simulink model "EMobility_V9"  (R2023b)
settings: Solver=VariableStepAuto  StartTime=0.0  StopTime=10.0  RelTol=1e-3
undefined symbols (not defined in the file): Ion, Lithium
libraries: spsSeriesRLCBranchLib x19, spsIdealSwitchLib x13, spsCurrentMeasurementLib x8, spsIGBTDiodeLib x7, spsVoltageMeasurementLib x7, simulink x3, spsPLLLib x3, spsDiodeLib x2, spsPWMGenerator2LevelLib x2, spsPWMGeneratorDCDCLib x2, spsPowerLib x2, spsRMSLib x2
settings Model: Creator=valentinaribeiro  LastModifiedBy=gradykirsch

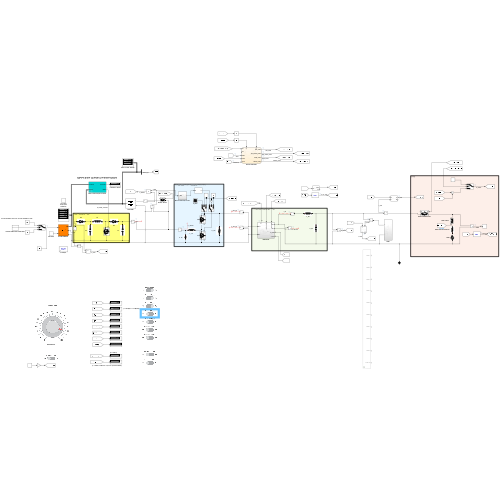
[thumbnail: Simulink's stored preview of the top-level diagram]
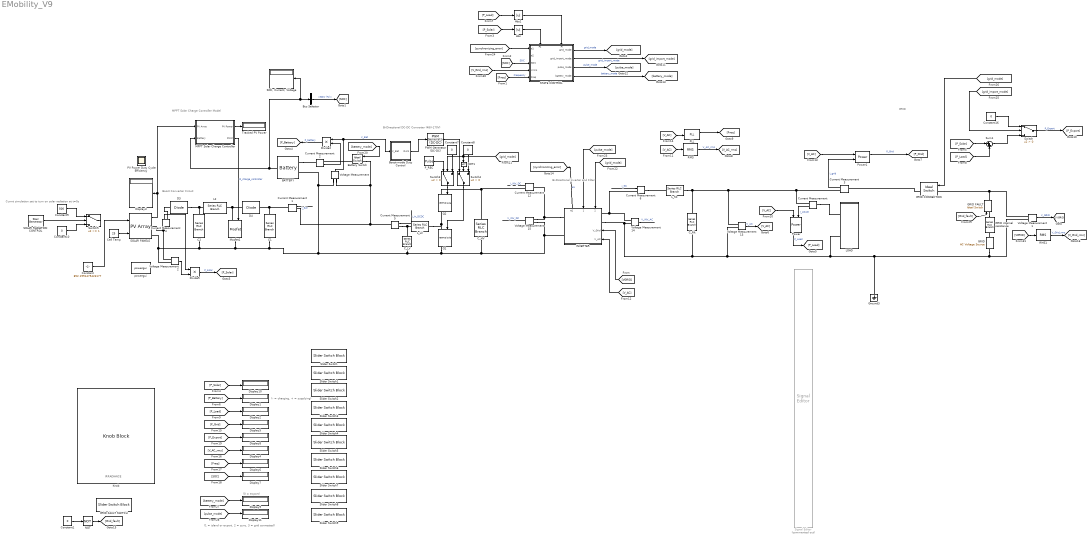
== system EMobility_V9 ==
  note: IRRADIANCE
  note: (- = charging, + = supplying)
  note: (0 = export)
  note: (1 = island or export, 2 = sync, 3 = grid connected)
  note: Bi-Directional Inverter and Filter
  note: GRID
  note: Boost Converter Circuit
  note: Bi-Directional DC-DC Converter (48V-170V)
  note: Currnt simulation set to turn on solar radiation at t=0s
  note: MPPT Solar Charge Controller Model
  " C1" : spsSeriesRLCBranchLib/Series RLC Branch  LConnTagsString=__new0  RConnTagsString=__new0  BranchType=C  Resistance=0.1  Inductance=1e-3  SetiL0=off  InitialCurrent=0  Capacitance=1  Setx0=off  InitialVoltage=0  Measurements=None
  Abs : Abs  SaturateOnIntegerOverflow=off
  Abs1 : Abs  SaturateOnIntegerOverflow=off
  BATTERY : spsBatteryLib/Battery  BatType=Lithium-Ion  ShowTempParam=off  ThermalPreset=no  ShowAgeParam=off  NomV=48  NomQ=80  SOC=89  Batt_Tr=30  PresetModel=on  MaxQ=80  MinV=36  FullV=55.8714  Dis_rate=34.7826  R=0.006  Normal_OP=72.3478  expZone="[51.8585      3.93043]"  current=[6.5 13 32.5]  Units=Time  Tci=20  NomT=20  T2=-30  MaxQ2=4.8  FullV2=7.1  Normal_OP2=5.655  expZone2="[6.58           1]"  Rca=0.6  ti=2000  Dp=0  Neq0=0  Tsim=1e6  Ta1=25  Qeol=5.4*0.9  Reol=0.013333*1.2  Char_age=[2.3478, 3]  Dis_age=[2.3478, 10]  N1=1500  N2=10500  N3=1000  N4=1400  Ta2=45  N5=950
      settings: LibrarySourceBlock=electricdrivelib/Extra Sources/Battery
  Battery Switch : spsIdealSwitchLib/Ideal Switch  Ron=0.001  Lon=0  IC=0  Rs=1e5  Cs=inf  Measurements=on
  Boost-mode Duty Control : Subsystem
  Bus Selector : BusSelector  OutputSignals=SOC (%)
  C2 : spsSeriesRLCBranchLib/Series RLC Branch  LConnTagsString=__new0  RConnTagsString=__new0  BranchType=C  Resistance=0.1  Inductance=1e-3  SetiL0=off  InitialCurrent=0  Capacitance=1000e-6  Setx0=off  InitialVoltage=0  Measurements=None
  C_HV : spsSeriesRLCBranchLib/Series RLC Branch  LConnTagsString=__new0  RConnTagsString=__new0  BranchType=C  Resistance=20  Inductance=159e-3  SetiL0=off  InitialCurrent=0  Capacitance=1.6e-3  Setx0=off  InitialVoltage=0  Measurements=None
  C_LV : spsSeriesRLCBranchLib/Series RLC Branch  LConnTagsString=__new0  RConnTagsString=__new0  BranchType=C  Resistance=20  Inductance=159e-3  SetiL0=off  InitialCurrent=0  Capacitance=0.5e-3  Setx0=off  InitialVoltage=0  Measurements=None
  C_filt : spsSeriesRLCBranchLib/Series RLC Branch  LConnTagsString=__new0  RConnTagsString=__new0  BranchType=C  Resistance=0  Inductance=1e-3  SetiL0=off  InitialCurrent=0  Capacitance=200e-6  Setx0=off  InitialVoltage=0  Measurements=None
  Cell Temp : Constant  Value=25
  Constant : Constant  Value=852.1991475423177
  Constant{1,7..8,10,16} (5 alike) : Constant  Value=0
  Constant9 : Constant  Value=500
  Current Measurement{,1..6,12} (8 alike) : spsCurrentMeasurementLib/Current Measurement  PhasorSimulation=off  OutputType=Complex  PSBequivalent=0
  D3 : spsDiodeLib/Diode  Ron=0.001  Lon=0  Vf=0.8  IC=0  UseSnubber=0  Rs=inf  Cs=0  Measurements=off
  D4 : spsDiodeLib/Diode  Ron=0.001  Lon=0  Vf=0.5  IC=0  UseSnubber=0  Rs=inf  Cs=0  Measurements=off
  Display{1..11} (11 alike) : Display
      Display7 settings: Decimation=1000
  Divide2 : Product  Inputs=**
  Divide5 : Product  Inputs=**
  GRID : spsACVoltageSourceLib/AC Voltage Source  Amplitude=170  Phase=0  Frequency=60  SampleTime=0  Measurements=None  BusType=swing  Pref=10e3  Qref=0  Qmin=-inf  Qmax=+inf
  GRID CONNECTION : spsIdealSwitchLib/Ideal Switch  Ron=0.001  Lon=0  IC=0  Rs=1e5  Cs=inf  Measurements=on
  GRID FAULT : spsIdealSwitchLib/Ideal Switch  Ron=0.001  Lon=0  IC=0  Rs=1e5  Cs=inf  Measurements=on
  GRID FAULT SWITCH : SliderSwitchBlock
      settings: Values={{'Off', 'On'}, [0 1]}
  GRID internal resistance : spsSeriesRLCBranchLib/Series RLC Branch  LConnTagsString=__new0  RConnTagsString=__new0  BranchType=R  Resistance=0.000001  Inductance=159e-3  SetiL0=off  InitialCurrent=0  Capacitance=100e-6  Setx0=off  InitialVoltage=0  Measurements=None
  Ground3 : spsGroundLib/Ground  LConnTagsString=a
  INVERTER : Subsystem
      settings: PortSchema="{\"entries\":[{\"content\":{\"sides\":[{\"content\":{\"connectorIds\":[\"LConn1\",\"LConn2\"]},\"type\":\"ConnectorPlacement.EquallySpacedRectSide\",\"uuid\":\"08b47f30-9f27-435b-83c4-c6fbe942e4e9\"},{\"content\":{\"connectorIds\":[\"RConn1\",\"RConn2\",\"In3\",\"In4\"],\"side\":\"RIGHT\"},\"type\":\"ConnectorPlacement.EquallySpacedRectSide\",\"uuid\":\"fbea0f57-7dc0-46de-be59-ba0dc15ef90e\"},{\"content\":{\"connectorIds\":[\"Out1\",\"In1\",\"In2\"],\"side\":\"TOP\"},\"type\":\"ConnectorPlacement.EquallySpacedRectSide\",\"uuid\":\"41f57134-76db-4888-b698-262c1208f49e\"}]},\"type\":\"ConnectorPlacement.EquallySpacedConnector\",\"uuid\":\"a2b9da51-a472-4525-b916-29c2121475f9\"}],\"packageUris\":[\"http://schema.mathworks.com/mf0/Connector/R2020b\"],\"version\":\"1.0\"}"
  Knob : KnobBlock  ScaleMax=1000
  L2 : spsSeriesRLCBranchLib/Series RLC Branch  LConnTagsString=__new0  RConnTagsString=__new0  BranchType=L  Resistance=1  Inductance=0.01  SetiL0=off  InitialCurrent=0  Capacitance=1e-6  Setx0=off  InitialVoltage=0  Measurements=None
  LOAD : Subsystem
  L_LV : spsSeriesRLCBranchLib/Series RLC Branch  LConnTagsString=__new0  RConnTagsString=__new0  BranchType=L  Resistance=0  Inductance=0.003  SetiL0=off  InitialCurrent=0  Capacitance=100e-6  Setx0=off  InitialVoltage=0  Measurements=None
  L_filt : spsSeriesRLCBranchLib/Series RLC Branch  LConnTagsString=__new0  RConnTagsString=__new0  BranchType=L  Resistance=0  Inductance=0.003  SetiL0=off  InitialCurrent=0  Capacitance=100e-6  Setx0=off  InitialVoltage=0  Measurements=None
  MPPT Solar Charge Controller : Subsystem  mask(MPPT Solar Charge Controller Block){dD=1e-6, BattCV=55.4, Fsw=1000}
      mask prompts: dD "MPPT Duty Cycle (delta) Step Size"; BattCV "Battery Charging Constant Voltage (V)"; Fsw "PWM Switching frequency (Hz):"
      mask help:
      | MPPT Solar Charge Controller Block
      | Developed by Rodney Tan (PhD)
      | Version 1.00 Oct 2019
      |
      | This block perform solar photovoltaic Maximum Power Point Tracking based on Perturbation & Observation algorithm and charge lead acid battery using three stage charging algorithm.
      mask Help:
      | <b><u>Block Setting</u></b>
      | 
      | <b>MPPT Duty Cycle Step Size</b>
      | Specify the MPPT duty cycle (delta) step size. Default value is 1e-5.
      | 
      | <b>Battery Charging Constant Voltage (V)</b>
      | Specify the battery charging constant voltage for absorption stage.
      | 
      | <b>PWM Switching Frequency (Hz)</b>
      | Specify the PWM switching frequency in Hz.
      mask TypeOptions Fsw:
      | PWM Generator
      | (DC-DC)/Fsw
  Mosfet1 : spsMosfetLib/Mosfet  Ron=0.02  Lon=0  Rd=0.01  Vfd=0  IC=0  Rs=1e5  Cs=inf  Measurements=off
  NOT : Logic  Operator=NOT  IconShape=distinctive  AllPortsSameDT=off  OutDataTypeStr=boolean
  NOT1 : Logic  Operator=NOT  IconShape=distinctive  AllPortsSameDT=off  OutDataTypeStr=boolean
  PLL : spsPLLLib/PLL  Fmin=45  Par_Init=[0, 60]  ParK=[180, 3200, 1]  TcD=1e-4  MaxRateChangeFreq=12  FilterCutOffFreq=25  Ts=0  AGC=on
      settings: LibrarySourceBlock=sps_lib/Control/PLL
  PV Power Duty Cycle Efficiency : Scope
      settings: Floating=on
  PWM Generator (DC-DC) : spsPWMGeneratorDCDCLib/PWM Generator (DC-DC)  Fsw=5000  Ts=0
  P_REC : DiscretePulseGenerator  PulseType=Time based  Period=1/5000  PulseWidth=26
  Power : spsPowerLib/Power  Freq=60  Vinit=[1, 0]  Iinit=[1, 0]  Ts=0
  Power1 : spsPowerLib/Power  Freq=60  Vinit=[1, 0]  Iinit=[1, 0]  Ts=0
  Q1 : spsIGBTDiodeLib/IGBT//Diode  Ron=1e-3  Rs=1e5  Cs=inf  Measurements=on
  Q2 : spsIGBTDiodeLib/IGBT//Diode  Ron=1e-3  Rs=1e5  Cs=inf  Measurements=on
  RMS : spsRMSLib/RMS  TrueRMS=on  Freq=60  RMSInit=120  Ts=0
  RMS1 : spsRMSLib/RMS  TrueRMS=on  Freq=60  RMSInit=120  Ts=0
  "SOC, Current, Voltage" : Display
  SOLAR PANELS : spsPVArrayLib/PV Array  Npar=8  Nser=10  PlotType=array @ 25 deg.C & specified irradiances  S_vec="[ 1000  800  600 400 200 ]"  Temp_C_vec="[ 45 25  ]"  ModuleName=Tesla Inc. SR24S3-2  PlotWhenSelected=off  Pm=23.4  Ncell=6  Voc=3.8  Isc=8.35  Vm=3  Im=7.8  beta_Voc_pc=-0.325  alpha_Isc_pc=0.048  beta_Voc=-0.01235  alpha_Isc=0.004008  IL=8.3755  I0=7.7166e-11  nI=0.97085  Rsh=23.4287  Rs=0.046227  RobustModel=off  RobustCellTemperature=313.3991  BAL=off  Tc=1e-6  Tfilter=1e-5
  SOLAR RADIATION CONTROL : spsStairGeneratorLib/Stair Generator  t=[0, 0.2, 0.4]  e=[1, 1, 1]  Ts=0
  STATE CONTROL : Stateflow chart  TreatAsAtomicUnit=on
      settings: PortSchema="{\"entries\":[{\"content\":{\"sides\":[{\"content\":{\"connectorIds\":[\"In3\",\"In5\",\"In6\",\"In4\",\"In7\"]},\"type\":\"ConnectorPlacement.EquallySpacedRectSide\",\"uuid\":\"b48b8e79-9223-4f44-9ca2-01abafb2610b\"},{\"content\":{\"connectorIds\":[\"Out1\",\"Out2\",\"Out3\",\"Out4\"],\"side\":\"RIGHT\"},\"type\":\"ConnectorPlacement.EquallySpacedRectSide\",\"uuid\":\"69043a30-cfac-4fa3-beb1-dafea7c61121\"},{\"content\":{\"connectorIds\":[\"In1\",\"In2\"],\"side\":\"TOP\"},\"type\":\"ConnectorPlacement.EquallySpacedRectSide\",\"uuid\":\"c5081c87-0412-4df0-923f-4518851b42d3\"}]},\"type\":\"ConnectorPlacement.EquallySpacedConnector\",\"uuid\":\"4eeccdef-121a-476a-b6e9-b0cda67e3776\"}],\"packageUris\":[\"http://schema.mathworks.com/mf0/Connector/R2020b\"],\"version\":\"1.0\"}"
  Signal Editor : SignalEditorBlockLib/Signal Editor  Commented=on  FileName=/Volumes/Extreme_SSD/MATLAB/loadsignal.mat  ActiveScenario=Scenario  ActiveSignal=Load 1  IsBus=off  OutputBusObjectStr=Bus: BusObject  SampleTime=0  Interpolate=off  ZeroCross=off  OutputAfterFinalValue=Setting to zero  Unit=inherit  PreserveSignalName=on  ApplySigPropsToAllScenarios=on  ApplySigPropsToAllSignals=off
  Slider Switch{,1..9} (10 alike) : SliderSwitchBlock
      settings: Values={{'Off', 'On'}, [0 1]}
  Sum1 : Sum  Inputs=|++
  Switch : Switch  Criteria=u2 > Threshold  SaturateOnIntegerOverflow=off  InputSameDT=off
  Switch3 : Switch  Criteria=u2 > Threshold  SaturateOnIntegerOverflow=off  InputSameDT=off
  Switch4 : Switch  Criteria=u2 > Threshold  SaturateOnIntegerOverflow=off  InputSameDT=off
  Switch5 : Switch  Threshold=1  SaturateOnIntegerOverflow=off  InputSameDT=off
  Tracked PV Power : Display
  Voltage Measurement{,1..2,13..15} (6 alike) : spsVoltageMeasurementLib/Voltage Measurement  PhasorSimulation=off  OutputType=Complex  PSBequivalent=0
  powergui : sps_lib/powergui  Priority=1  SimulationMode=Discrete  SampleTime=1/1e5  frequency=60  Iterations=50  frequencyindice=0  Pbase=100e6  ErrMax=1e-4  UnitsV=kV  UnitsW=MW  buscounter=0  FunctionMessages=off  echomessages=off  EnableUseOfTLC=off  CurrentSourceSwitches=off  DisableSnubberDevices=off  DisableRonSwitches=off  DisableVfSwitches=off  DisplayEquations=off  AutomaticDiscreteSolvers=off  SolverType=Tustin/Backward Euler (TBE)  Interpol=off  ExternalGateDelay=off  methode=off  Ts=100  x0status=blocks  SPID=off  SwTol=0  HookPort=off  NonlinearTolerance=1e-4  nMaxIteration=100  ContinueOnMaxIteration=off  RestoreLinks=warning  ResistiveCurrentMeasurement=off  Frange=[0:2:500]  Ylog=off  Xlog=on  ShowGrid=off  save=off  variable=ZData  structure=0  ZoomFFT=off  StartTime=0.0  cycles=1  DisplayStyle=1  fundamental=60  FreqAxis=off  MaxFrequency=1000  frequencyindicesteady=1  RmsSteady=1  display=off
  wires:
  Voltage Measurement15/1 -> ?  "V_INV_DC"
  SOLAR PANELS/1 -> MPPT Solar Charge Controller/1(PV Array), Display3/1
  RMS/1 -> [V_AC_rms]  "V_AC_rms"
  INVERTER/1(e1) -> [synchronizing_error]  "e1"
  Divide2/1 -> [P_Battery]  "P_battery"
  P_REC/1 -> Switch3/1
  NOT1/1 -> Switch4/2
  Current Measurement/1 -> Power/2  "I_LOAD"
  Voltage Measurement14/1 -> ?  "V_INV_AC"
  STATE CONTROL/3(pulse_mode) -> [pulse_mode]  "pulse_mode"
  Voltage Measurement13/1 -> [V_AC]  "V_AC"
  Current Measurement2/1 -> Divide2/2
  Constant7/1 -> Switch3/3
  Voltage Measurement1/1 -> [VGRID]  "V_GRID"
  BATTERY/1 -> Bus Selector/1, "SOC, Current, Voltage"/1, MPPT Solar Charge Controller/2(Battery)
  Constant10/1 -> Switch5/3
  SOLAR RADIATION CONTROL/1 -> Switch5/2
  Switch3/1 -> Q2/1
  Switch4/1 -> Q1/1
  PWM Generator (DC-DC)/1 -> Switch4/1
  MPPT Solar Charge Controller/1(PV Power) -> Tracked PV Power/1
  Cell Temp/1 -> SOLAR PANELS/2
  MPPT Solar Charge Controller/2(PWM) -> Mosfet1/1  "D_charge_controller"
  Current Measurement12/1 -> ?  "I_INV_DC"
  Constant9/1 -> Switch5/1
  PLL/1 -> [Freq]
  Voltage Measurement/1 -> Divide2/1, Boost-mode Duty Control/1(V_Bat)  "V_Bat"
  [VGRID] -> INVERTER/3(V_Grid)
  Constant8/1 -> Switch4/3
  STATE CONTROL/1(grid_mode) -> [grid_mode]  "grid_mode"
  Bus Selector/1 -> [SOC]  "<SOC (%)>"
  Current Measurement3/1 -> Power1/2  "I_grid"
  Divide5/1 -> [P_Solar]  "P_solar"
  Voltage Measurement2/1 -> Divide5/2
  Current Measurement4/1 -> Divide5/1
  Abs1/1 -> STATE CONTROL/2(Pl)
  Abs/1 -> STATE CONTROL/1(Ps)
  Power1/1 -> [P_Grid]  "P_Grid"
  Power/1 -> [P_Load]  "P_Load"
  STATE CONTROL/4(battery_mode) -> [battery_mode]  "battery_mode"
  STATE CONTROL/2(grid_import_mode) -> [grid_import_mode]  "grid_import_mode"
  Current Measurement5/1 -> ?  "i_in_DCDC"
  Current Measurement6/1 -> ?  "I_filt"
  Switch/1 -> [P_Export]  "P_Export"
  Sum1/1 -> Switch/3
  Constant16/1 -> Switch/1
  [P_Solar] -> Abs/1
  [P_Solar] -> Display10/1
  [P_Solar] -> Sum1/1
  Boost-mode Duty Control/1(Out1) -> PWM Generator (DC-DC)/1
  Current Measurement1/1 -> ?  "I_Sun"
  [P_Battery] -> Display1/1
  [P_Load] -> Abs1/1
  [P_Load] -> Sum1/2
  [P_Load] -> Display2/1
  [V_AC] -> Power/1
  [V_AC] -> RMS/1
  [V_AC] -> INVERTER/4(V_AC)
  [V_AC] -> Power1/1
  [V_AC] -> PLL/1
  [P_Grid] -> Display5/1
  [Freq] -> Display6/1
  [V_AC_rms] -> Display4/1
  [Freq] -> STATE CONTROL/7(Freq)  "Frequency"
  [SOC] -> STATE CONTROL/6(SOC)  "SOC"
  [SOC] -> Display7/1
  [P_Export] -> Display8/1
  [battery_mode] -> Battery Switch/1
  [grid_mode] -> NOT1/1, Switch3/2
  [grid_mode] -> INVERTER/2(grid_mode)
  [pulse_mode] -> INVERTER/1(pulse_mode)
  [synchronizing_error] -> STATE CONTROL/3(e1)
  [grid_import_mode] -> Switch/2
  [grid_mode] -> GRID CONNECTION/1
  [pulse_mode] -> Display11/1
  [battery_mode] -> Display9/1
  Constant/1 -> SOLAR PANELS/1
  [Grid_fault] -> GRID FAULT/1
  Constant1/1 -> NOT/1
  NOT/1 -> [Grid_fault]
  [V_Grid_rms] -> STATE CONTROL/4(Vrms)
  RMS1/1 -> [V_Grid_rms]  "V_Grid_rms"
  [VGRID] -> RMS1/1
  connections:
  C_LV/RConn1 -- Voltage Measurement/LConn2 -- BATTERY/LConn2 -- " C1"/RConn1 -- Mosfet1/RConn1 -- SOLAR PANELS/RConn2 -- Voltage Measurement2/LConn2 -- C2/RConn1 -- Q1/RConn1 -- C_HV/RConn1 -- Voltage Measurement15/LConn2 -- INVERTER/LConn2
  Current Measurement1/RConn1 -- Battery Switch/LConn1 -- Voltage Measurement/LConn1 -- Current Measurement5/LConn1
  Voltage Measurement1/LConn1 -- GRID FAULT/RConn1 -- GRID CONNECTION/LConn1
  L2/LConn1 -- C2/LConn1 -- D3/RConn1
  L_filt/RConn1 -- Current Measurement/RConn1 -- Current Measurement3/RConn1 -- Voltage Measurement13/LConn1 -- C_filt/LConn1
  Voltage Measurement13/LConn2 -- GRID/LConn1 -- Voltage Measurement1/LConn2 -- Ground3/LConn1 -- LOAD/LConn2 -- INVERTER/RConn2 -- Voltage Measurement14/LConn2 -- C_filt/RConn1
  INVERTER/LConn1 -- Current Measurement12/LConn1 -- Voltage Measurement15/LConn1
  L_LV/RConn1 -- Q2/RConn1 -- Q1/LConn1
  Mosfet1/LConn1 -- L2/RConn1 -- D4/LConn1
  C_HV/LConn1 -- Q2/LConn1 -- Current Measurement12/RConn1
  Voltage Measurement14/LConn1 -- Current Measurement6/RConn1 -- INVERTER/RConn1
  GRID/RConn1 -- GRID internal resistance/LConn1
  BATTERY/LConn1 -- Current Measurement2/LConn1
  GRID CONNECTION/RConn1 -- Current Measurement3/LConn1
  " C1"/LConn1 -- Current Measurement1/LConn1 -- D4/RConn1
  Current Measurement4/LConn1 -- Voltage Measurement2/LConn1 -- SOLAR PANELS/RConn1
  D3/LConn1 -- Current Measurement4/RConn1
  Battery Switch/RConn1 -- Current Measurement2/RConn1
  L_LV/LConn1 -- Current Measurement5/RConn1 -- C_LV/LConn1
  Current Measurement6/LConn1 -- L_filt/LConn1
  Current Measurement/LConn1 -- LOAD/LConn1
  GRID FAULT/LConn1 -- GRID internal resistance/RConn1

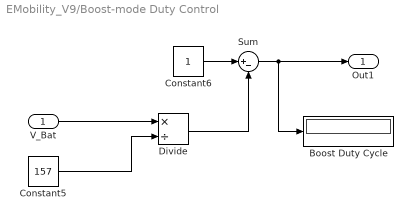
== system EMobility_V9/Boost-mode Duty Control ==
  V_Bat : Inport
  Boost Duty Cycle : Display
  Constant5 : Constant  Value=157
  Constant6 : Constant
  Divide : Product  Inputs=*/
  Sum : Sum  Inputs=|+-
  Out1 : Outport
  wires:
  Divide/1 -> Sum/2
  Constant6/1 -> Sum/1
  V_Bat/1 -> Divide/1
  Constant5/1 -> Divide/2
  Sum/1 -> Out1/1, Boost Duty Cycle/1

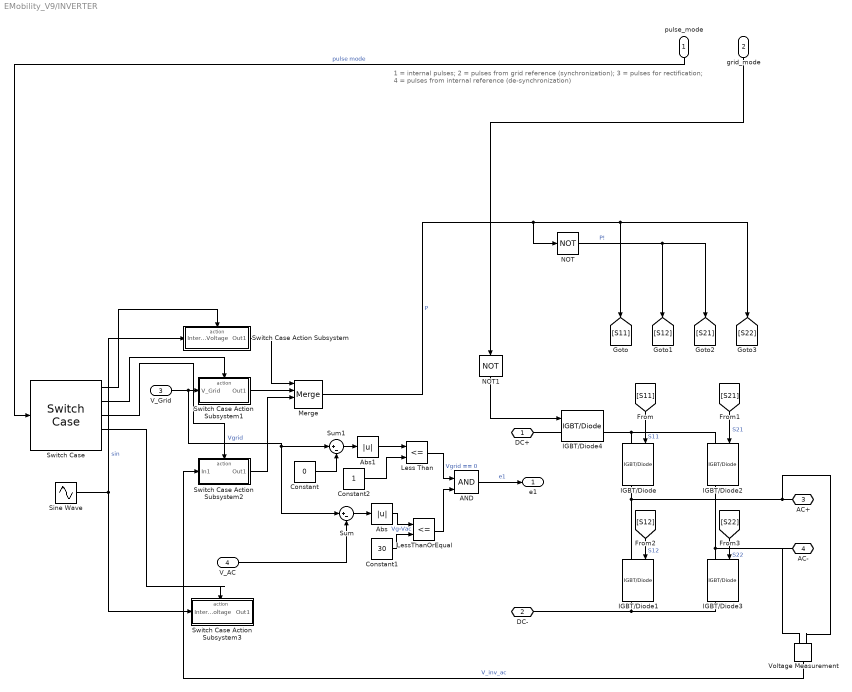
== system EMobility_V9/INVERTER ==
  note: 1 = internal pulses; 2 = pulses from grid reference (synchronization); 3 = pulses for rectification; 4 = pulses from internal reference (de-synchronization)
  pulse_mode : Inport
  grid_mode : Inport  Port=2
  V_Grid : Inport  Port=3
  V_AC : Inport  Port=4
  AND : Logic  IconShape=distinctive  AllPortsSameDT=off  OutDataTypeStr=boolean
  Abs : Abs  SaturateOnIntegerOverflow=off
  Abs1 : Abs  SaturateOnIntegerOverflow=off
  Constant : Constant  Value=0
  Constant1 : Constant  Value=30
  Constant2 : Constant
  IGBT/Diode{,1..4} (5 alike) : spsIGBTDiodeLib/IGBT//Diode  Ron=1e-3  Rs=1e5  Cs=inf  Measurements=on
  Less Than : RelationalOperator  Operator=<=  OutDataTypeStr=boolean  RndMeth=Simplest  InputSameDT=off
  LessThanOrEqual : RelationalOperator  Operator=<=  OutDataTypeStr=boolean  RndMeth=Simplest  InputSameDT=off
  Merge : Merge  Inputs=4
  NOT : Logic  Operator=NOT  IconShape=distinctive  AllPortsSameDT=off  OutDataTypeStr=boolean
  NOT1 : Logic  Operator=NOT  IconShape=distinctive  AllPortsSameDT=off  OutDataTypeStr=boolean
  Sine Wave : Sin  Frequency=60*2*pi  Phase=pi/2  SampleTime=0
  Sum : Sum  Inputs=|+-
  Sum1 : Sum  Inputs=|+-
  Switch Case : SwitchCase  CaseConditions={1,2,3,4}
  Switch Case Action Subsystem : Subsystem  TreatAsAtomicUnit=on
  Switch Case Action Subsystem1 : Subsystem  TreatAsAtomicUnit=on
  Switch Case Action Subsystem2 : Subsystem  TreatAsAtomicUnit=on
  Switch Case Action Subsystem3 : Subsystem  TreatAsAtomicUnit=on
  Voltage Measurement : spsVoltageMeasurementLib/Voltage Measurement  PhasorSimulation=off  OutputType=Complex  PSBequivalent=0
  DC+ : PMIOPort  Side=Left
  DC- : PMIOPort  Port=2  Side=Left
  AC+ : PMIOPort  Port=3  Side=Right
  AC- : PMIOPort  Port=4  Side=Right
  e1 : Outport
  wires:
  [S11] -> IGBT/Diode/1  "S11"
  [S21] -> IGBT/Diode2/1  "S21"
  [S12] -> IGBT/Diode1/1  "S12"
  [S22] -> IGBT/Diode3/1  "S22"
  Merge/1 -> NOT/1, [S11], [S22]  "P"
  NOT/1 -> [S21], [S12]  "P!"
  Voltage Measurement/1 -> Switch Case Action Subsystem2/1(In1)  "V_inv_ac"
  pulse_mode/1 -> Switch Case/1  "pulse mode"
  NOT1/1 -> IGBT/Diode4/1
  V_Grid/1 -> Sum1/1, Sum/1, Switch Case Action Subsystem1/1(V_Grid)  "Vgrid"
  Switch Case/1 -> Switch Case Action Subsystem/Action
  Switch Case/2 -> Switch Case Action Subsystem1/Action
  Switch Case/3 -> Switch Case Action Subsystem2/Action
  Switch Case Action Subsystem/1(Out1) -> Merge/1
  Switch Case Action Subsystem1/1(Out1) -> Merge/2
  Switch Case Action Subsystem2/1(Out1) -> Merge/3
  grid_mode/1 -> NOT1/1
  Sum/1 -> Abs/1
  Less Than/1 -> AND/1  "Vgrid == 0"
  AND/1 -> e1/1  "e1"
  Abs/1 -> LessThanOrEqual/1  "Vg-Vac"
  Constant1/1 -> LessThanOrEqual/2
  LessThanOrEqual/1 -> AND/2
  Constant/1 -> Sum1/2
  Constant2/1 -> Less Than/2
  Sum1/1 -> Abs1/1
  Abs1/1 -> Less Than/1
  V_AC/1 -> Sum/2
  Switch Case/4 -> Switch Case Action Subsystem3/Action
  Sine Wave/1 -> Switch Case Action Subsystem3/1(Internal Voltage), Switch Case Action Subsystem/1(Internal Voltage)  "sin"
  connections:
  AC+/RConn1 -- IGBT/Diode1/LConn1 -- IGBT/Diode/RConn1 -- Voltage Measurement/LConn1
  IGBT/Diode1/RConn1 -- DC-/RConn1 -- IGBT/Diode3/RConn1
  IGBT/Diode3/LConn1 -- Voltage Measurement/LConn2 -- AC-/RConn1 -- IGBT/Diode2/RConn1
  IGBT/Diode/LConn1 -- IGBT/Diode2/LConn1 -- IGBT/Diode4/RConn1
  IGBT/Diode4/LConn1 -- DC+/RConn1

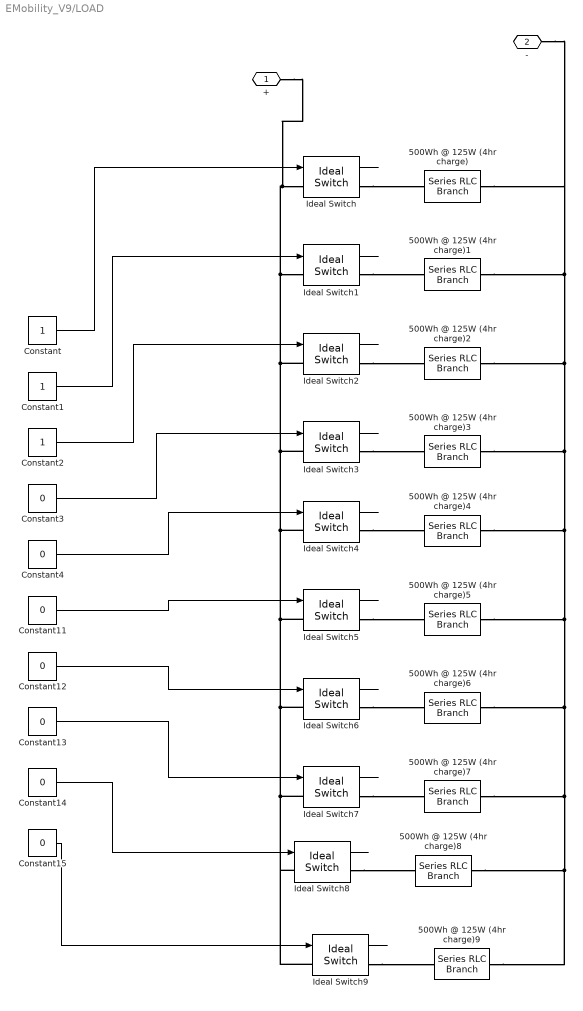
== system EMobility_V9/LOAD ==
  500Wh @ 125W (4hr charge){,1..9} (10 alike) : spsSeriesRLCBranchLib/Series RLC Branch  LConnTagsString=__new0  RConnTagsString=__new0  BranchType=R  Resistance=120  Inductance=1e-3  SetiL0=off  InitialCurrent=0  Capacitance=80e-6  Setx0=off  InitialVoltage=0  Measurements=None
  Constant : Constant
  Constant1 : Constant
  Constant{3..4,11..15} (7 alike) : Constant  Value=0
  Constant2 : Constant
  Ideal Switch{,1..9} (10 alike) : spsIdealSwitchLib/Ideal Switch  Ron=0.001  Lon=0  IC=0  Rs=1e5  Cs=inf  Measurements=on
  + : PMIOPort  Side=Left
  - : PMIOPort  Port=2  Side=Left
  wires:
  Ideal Switch2/1 -> ?
  Ideal Switch/1 -> ?
  Ideal Switch4/1 -> ?
  Constant12/1 -> Ideal Switch6/1
  Constant14/1 -> Ideal Switch8/1
  Constant11/1 -> Ideal Switch5/1
  Constant/1 -> Ideal Switch/1
  Constant3/1 -> Ideal Switch3/1
  Constant2/1 -> Ideal Switch2/1
  Ideal Switch9/1 -> ?
  Constant13/1 -> Ideal Switch7/1
  Ideal Switch3/1 -> ?
  Ideal Switch7/1 -> ?
  Ideal Switch1/1 -> ?
  Ideal Switch6/1 -> ?
  Constant1/1 -> Ideal Switch1/1
  Ideal Switch8/1 -> ?
  Constant15/1 -> Ideal Switch9/1
  Constant4/1 -> Ideal Switch4/1
  Ideal Switch5/1 -> ?
  connections:
  Ideal Switch6/RConn1 -- 500Wh @ 125W (4hr charge)6/LConn1
  Ideal Switch2/RConn1 -- 500Wh @ 125W (4hr charge)2/LConn1
  Ideal Switch/RConn1 -- 500Wh @ 125W (4hr charge)/LConn1
  Ideal Switch1/RConn1 -- 500Wh @ 125W (4hr charge)1/LConn1
  Ideal Switch4/RConn1 -- 500Wh @ 125W (4hr charge)4/LConn1
  Ideal Switch5/RConn1 -- 500Wh @ 125W (4hr charge)5/LConn1
  Ideal Switch7/RConn1 -- 500Wh @ 125W (4hr charge)7/LConn1
  Ideal Switch9/RConn1 -- 500Wh @ 125W (4hr charge)9/LConn1
  Ideal Switch3/RConn1 -- 500Wh @ 125W (4hr charge)3/LConn1
  Ideal Switch8/RConn1 -- 500Wh @ 125W (4hr charge)8/LConn1
  500Wh @ 125W (4hr charge)9/RConn1 -- -/RConn1 -- 500Wh @ 125W (4hr charge)/RConn1 -- 500Wh @ 125W (4hr charge)1/RConn1 -- 500Wh @ 125W (4hr charge)2/RConn1 -- 500Wh @ 125W (4hr charge)3/RConn1 -- 500Wh @ 125W (4hr charge)4/RConn1 -- 500Wh @ 125W (4hr charge)5/RConn1 -- 500Wh @ 125W (4hr charge)6/RConn1 -- 500Wh @ 125W (4hr charge)7/RConn1 -- 500Wh @ 125W (4hr charge)8/RConn1
  Ideal Switch4/LConn1 -- Ideal Switch6/LConn1 -- Ideal Switch9/LConn1 -- Ideal Switch8/LConn1 -- Ideal Switch7/LConn1 -- Ideal Switch5/LConn1 -- +/RConn1 -- Ideal Switch/LConn1 -- Ideal Switch1/LConn1 -- Ideal Switch2/LConn1 -- Ideal Switch3/LConn1

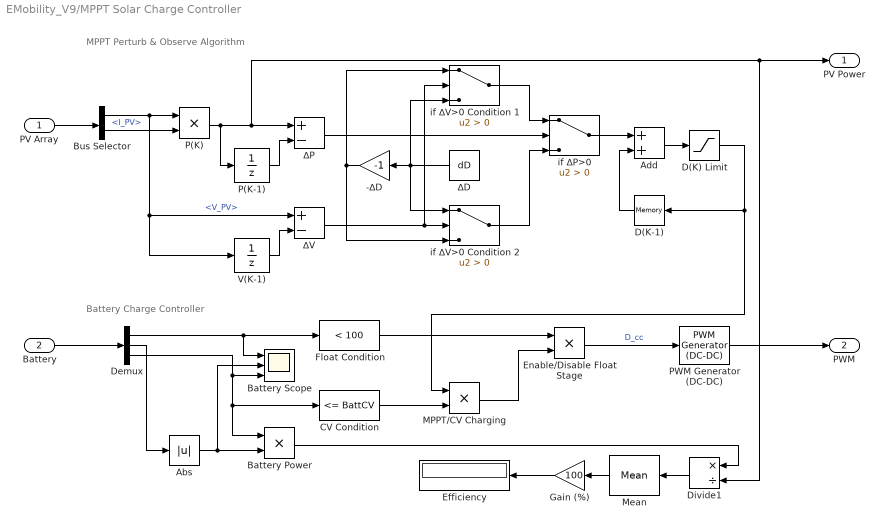
== system EMobility_V9/MPPT Solar Charge Controller ==
  note: Battery Charge Controller
  note: MPPT Perturb & Observe Algorithm
  PV Array : Inport
  Battery : Inport  Port=2
  -∆D : Gain  Gain=-1
  Abs : Abs  SaturateOnIntegerOverflow=off
  Add : Sum
  Battery Power : Product
  Battery Scope : Scope  NumInputPorts=3
  Bus Selector : BusSelector  OutputSignals=V_PV,I_PV
  CV Condition : simulink/Logic and Bit Operations/Compare To Constant  relop=<=  const=BattCV  OutDataTypeStr=boolean
  D(K) Limit : Saturate  UpperLimit=0.6  LowerLimit=0.4
  D(K-1) : Memory  InitialCondition=0.5  InheritSampleTime=on  LinearizeMemory=on  LinearizeAsDelay=on
  Demux : Demux  Outputs=3
  Divide1 : Product  Inputs=*/
  Efficiency : Display
  Enable/Disable Float Stage : Product
  Float Condition : simulink/Logic and Bit Operations/Compare To Constant  relop=<  const=100  OutDataTypeStr=boolean
  Gain (%) : Gain  Gain=100
  MPPT/CV Charging : Product
  Mean : spsMeanLib/Mean  Freq=1  Vinit=0  Ts=0
  P(K) : Product
  P(K-1) : UnitDelay  SampleTime=-1  HasFrameUpgradeWarning=on
  PWM Generator (DC-DC) : spsPWMGeneratorDCDCLib/PWM Generator (DC-DC)  Fsw=Fsw  Ts=0
  V(K-1) : UnitDelay  SampleTime=-1  HasFrameUpgradeWarning=on
  if ∆P>0 : Switch  Criteria=u2 > Threshold  SaturateOnIntegerOverflow=off  InputSameDT=off
  if ∆V>0 Condition 1 : Switch  Criteria=u2 > Threshold  SaturateOnIntegerOverflow=off  InputSameDT=off
  if ∆V>0 Condition 2 : Switch  Criteria=u2 > Threshold  SaturateOnIntegerOverflow=off  InputSameDT=off
  ∆D : Constant  Value=dD
  ∆P : Sum  Inputs=+-
  ∆V : Sum  Inputs=+-
  PV Power : Outport  VectorParamsAs1DForOutWhenUnconnected=off
  PWM : Outport  Port=2  VectorParamsAs1DForOutWhenUnconnected=off
  wires:
  P(K)/1 -> ∆P/1, Divide1/2, PV Power/1, P(K-1)/1
  if ∆V>0 Condition 1/1 -> if ∆P>0/1
  ∆P/1 -> if ∆P>0/2
  P(K-1)/1 -> ∆P/2
  V(K-1)/1 -> ∆V/2
  ∆V/1 -> if ∆V>0 Condition 2/2, if ∆V>0 Condition 1/2
  Add/1 -> D(K) Limit/1
  if ∆V>0 Condition 2/1 -> if ∆P>0/3
  D(K-1)/1 -> Add/2
  ∆D/1 -> if ∆V>0 Condition 2/1, -∆D/1, if ∆V>0 Condition 1/3
  -∆D/1 -> if ∆V>0 Condition 2/3, if ∆V>0 Condition 1/1
  PWM Generator (DC-DC)/1 -> PWM/1
  Enable/Disable Float Stage/1 -> PWM Generator (DC-DC)/1  "D_cc"
  Float Condition/1 -> Enable/Disable Float Stage/1
  CV Condition/1 -> MPPT/CV Charging/2
  Battery/1 -> Demux/1
  Demux/3 -> Battery Scope/3, CV Condition/1, Battery Power/1
  Demux/1 -> Float Condition/1, Battery Scope/1
  MPPT/CV Charging/1 -> Enable/Disable Float Stage/2
  Demux/2 -> Abs/1
  Divide1/1 -> Mean/1
  Mean/1 -> Gain (%)/1
  Abs/1 -> Battery Scope/2, Battery Power/2
  Bus Selector/2 -> P(K)/2  "<I_PV>"
  Battery Power/1 -> Divide1/1
  Bus Selector/1 -> ∆V/1, V(K-1)/1, P(K)/1  "<V_PV>"
  PV Array/1 -> Bus Selector/1
  if ∆P>0/1 -> Add/1
  D(K) Limit/1 -> D(K-1)/1, MPPT/CV Charging/1
  Gain (%)/1 -> Efficiency/1

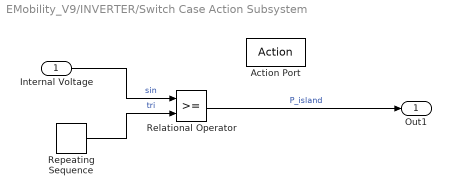
== system EMobility_V9/INVERTER/Switch Case Action Subsystem ==
  Internal Voltage : Inport
  Action Port : ActionPort  ActionPortLabel=case [ 1 ]:
  Relational Operator : RelationalOperator  OutDataTypeStr=boolean  RndMeth=Simplest  InputSameDT=off
  Repeating Sequence : simulink/Sources/Repeating Sequence  rep_seq_t=[0 0.5/5000 1/5000]  rep_seq_y=[-1 1 -1]
  Out1 : Outport
  wires:
  Relational Operator/1 -> Out1/1  "P_island"
  Internal Voltage/1 -> Relational Operator/1  "sin"
  Repeating Sequence/1 -> Relational Operator/2  "tri"

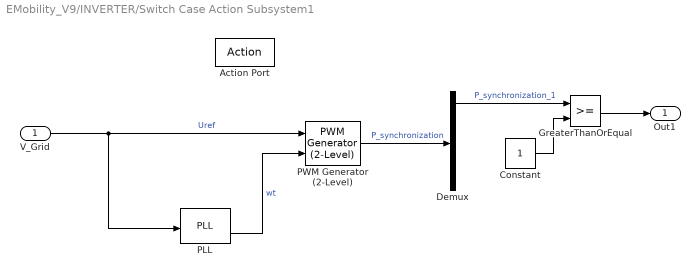
== system EMobility_V9/INVERTER/Switch Case Action Subsystem1 ==
  V_Grid : Inport
  Action Port : ActionPort  ActionPortLabel=case [ 2 ]:
  Constant : Constant
  Demux : Demux
  GreaterThanOrEqual : RelationalOperator  OutDataTypeStr=boolean  RndMeth=Simplest  InputSameDT=off
  PLL : spsPLLLib/PLL  Fmin=45  Par_Init=[0, 60]  ParK=[180, 3200, 1]  TcD=1e-4  MaxRateChangeFreq=12  FilterCutOffFreq=25  Ts=0  AGC=on
      settings: LibrarySourceBlock=sps_lib/Control/PLL
  PWM Generator (2-Level) : spsPWMGenerator2LevelLib/PWM Generator (2-Level)  ModulatorType=Single-phase full-bridge (4 pulses)  ModulatorMode=Synchronized  Fc=27*60  Pc=90  nF=83  MinMax="[ -185  185 ]"  SamplingTechnique=Natural  ModulatingSignals=off  m=0.8  Freq=60  Phase=0  Ts=0  ShowCarrierOutport=off
  Out1 : Outport
  wires:
  PLL/2 -> PWM Generator (2-Level)/2  "wt"
  PWM Generator (2-Level)/1 -> Demux/1  "P_synchronization"
  Demux/1 -> GreaterThanOrEqual/1  "P_synchronization_1"
  GreaterThanOrEqual/1 -> Out1/1
  Constant/1 -> GreaterThanOrEqual/2
  V_Grid/1 -> PWM Generator (2-Level)/1, PLL/1  "Uref"

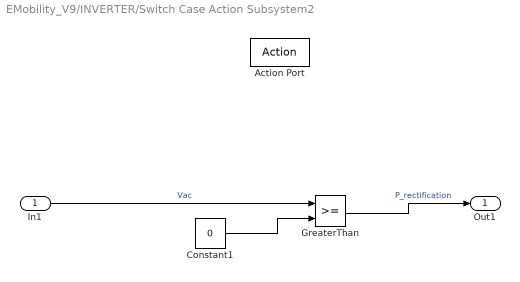
== system EMobility_V9/INVERTER/Switch Case Action Subsystem2 ==
  In1 : Inport
  Action Port : ActionPort  ActionPortLabel=case [ 3 ]:
  Constant1 : Constant  Value=0
  GreaterThan : RelationalOperator  OutDataTypeStr=boolean  RndMeth=Simplest  InputSameDT=off
  Out1 : Outport
  wires:
  In1/1 -> GreaterThan/1  "Vac"
  Constant1/1 -> GreaterThan/2
  GreaterThan/1 -> Out1/1  "P_rectification"

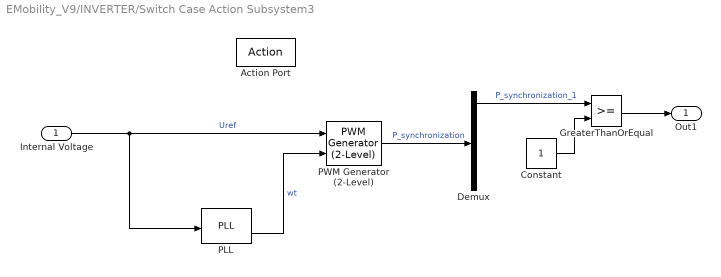
== system EMobility_V9/INVERTER/Switch Case Action Subsystem3 ==
  Internal Voltage : Inport
  Action Port : ActionPort  ActionPortLabel=case [ 4 ]:
  Constant : Constant
  Demux : Demux
  GreaterThanOrEqual : RelationalOperator  OutDataTypeStr=boolean  RndMeth=Simplest  InputSameDT=off
  PLL : spsPLLLib/PLL  Fmin=45  Par_Init=[0, 60]  ParK=[180, 3200, 1]  TcD=1e-4  MaxRateChangeFreq=12  FilterCutOffFreq=25  Ts=0  AGC=on
      settings: LibrarySourceBlock=sps_lib/Control/PLL
  PWM Generator (2-Level) : spsPWMGenerator2LevelLib/PWM Generator (2-Level)  ModulatorType=Single-phase full-bridge (4 pulses)  ModulatorMode=Synchronized  Fc=27*60  Pc=90  nF=83  MinMax="[ -185  185 ]"  SamplingTechnique=Natural  ModulatingSignals=off  m=0.8  Freq=60  Phase=0  Ts=0  ShowCarrierOutport=off
  Out1 : Outport
  wires:
  PLL/2 -> PWM Generator (2-Level)/2  "wt"
  PWM Generator (2-Level)/1 -> Demux/1  "P_synchronization"
  Demux/1 -> GreaterThanOrEqual/1  "P_synchronization_1"
  GreaterThanOrEqual/1 -> Out1/1
  Constant/1 -> GreaterThanOrEqual/2
  Internal Voltage/1 -> PWM Generator (2-Level)/1, PLL/1  "Uref"

== stateflow chart EMobility_V9/STATE CONTROL ==
  state Grid_Export
    grid_mode = 0;
    pulse_mode = 1;
    battery_mode = 0;
    grid_import_mode = 0;
  state Synchronize
    grid_mode = 0;
    pulse_mode = 2;
    battery_mode = 1;
    grid_import_mode = 1;
  state Grid_Connected
    grid_mode = 1;
    pulse_mode = 3;
    battery_mode = 1;
    grid_import_mode = 1;
  state Island
    grid_mode = 0;
    pulse_mode = 1;
    battery_mode = 1;
    grid_import_mode = 1;
  state De_synchronize [commented out]
    grid_mode = 1;
    pulse_mode = 4;
    battery_mode = 1;
    grid_import_mode = 1;
  Island -> Synchronize [order 3] : [Ps>m&&Pl>n&&(Ps-Pl)<k&&SOC<20&&Vrms>114&&Vrms<126]
  Island -> Synchronize [order 2] : [SOC < 20&&Ps<m&&Pl>n&&Vrms>114&&Vrms<126]
  Island -> Grid_Export [order 1] : [after(0.1,sec)&&Ps>m&&(Ps-Pl)>k&&SOC>80]
  Synchronize -> Grid_Connected : [e1 == 1&&SOC<20]
  Grid_Export -> De_synchronize [commented out] : [Freq>65||Freq<45]
  Grid_Export -> De_synchronize [commented out] : [(Ps-Pl)<k]
  Grid_Export -> Island : [(Ps-Pl)<k]
  Grid_Connected -> Island [order 1] : [SOC > 80]
  (default) -> Island
  Grid_Connected -> Island [order 2] : [Freq<45||Freq>65]
  Grid_Connected -> Island [order 3] : [after(0.1,sec)&&(Vrms<114||Vrms>126)]
  Grid_Connected -> De_synchronize [commented out] : [Freq<45||Freq>65]
  Grid_Connected -> De_synchronize [commented out] : [SOC > 80]
  De_synchronize -> Island [commented out] : [e2 < Ki]
  data: Ps input; Pl input; e1 input; Vrms input; e2 input; SOC input; grid_mode output; grid_import_mode output; pulse_mode output; Kg constant double =10; Ki constant double =10; Freq input; k constant double =500; n constant double =1; m constant double =5; battery_mode output
